simulink model "linearExtendedStateObserverModel"  (R2021a)
settings: Solver=VariableStepAuto  StartTime=0.0  StopTime=10.0  RelTol=1e-3
settings Model: Creator=krzys  LastModifiedBy=krzys

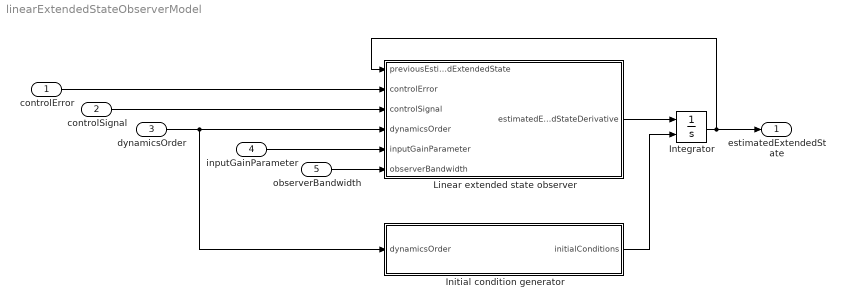
== system linearExtendedStateObserverModel ==
  controlError : Inport
  controlSignal : Inport  Port=2
  dynamicsOrder : Inport  Port=3
  inputGainParameter : Inport  Port=4
  observerBandwidth : Inport  Port=5
  Initial condition generator : MATLAB Function  TreatAsAtomicUnit=on
  Integrator : Integrator  InitialConditionSource=external
  Linear extended state observer : MATLAB Function  TreatAsAtomicUnit=on
  estimatedExtendedState : Outport
  wires:
  controlError/1 -> Linear extended state observer/2(controlError)
  controlSignal/1 -> Linear extended state observer/3(controlSignal)
  Linear extended state observer/1(estimatedExtendedStateDerivative) -> Integrator/1
  dynamicsOrder/1 -> Initial condition generator/1(dynamicsOrder), Linear extended state observer/4(dynamicsOrder)
  inputGainParameter/1 -> Linear extended state observer/5(inputGainParameter)
  observerBandwidth/1 -> Linear extended state observer/6(observerBandwidth)
  Initial condition generator/1(initialConditions) -> Integrator/2
  Integrator/1 -> Linear extended state observer/1(previousEstimatedExtendedState), estimatedExtendedState/1

== matlab function linearExtendedStateObserverModel/Initial condition generator ==
  data: dynamicsOrder input; initialConditions output
function initialConditions = fcn(dynamicsOrder)
    initialConditions = zeros(dynamicsOrder,1);
end

== matlab function linearExtendedStateObserverModel/Linear extended state observer ==
  data: previousEstimatedExtendedState input; controlError input; estimatedExtendedStateDerivative output; controlSignal input; dynamicsOrder input; inputGainParameter input; observerBandwidth input
function estimatedExtendedStateDerivative = fcn(previousEstimatedExtendedState,...
        controlError,...
        controlSignal,...
        dynamicsOrder,...
        inputGainParameter,...
        observerBandwidth)
    
    A = calculateObserverStateMatrix(dynamicsOrder);
    B = calculateObserverInputMatrix(inputGainParameter, dynamicsOrder);
    L = calculateObserverGainVector(observerBandwidth, dynamicsOrder);
    
    estimatedExtendedStateDerivative = A * previousEstimatedExtendedState +...
        B * controlSignal +...
        L * (controlError - previousEstimatedExtendedState(1));
end

function observerStateMatrix = calculateObserverStateMatrix(dynamicsOrder)
    observerStateMatrix = [zeros(dynamicsOrder,1), eye(dynamicsOrder);...
        zeros(1,dynamicsOrder+1)];
end

function observerInputMatrix = calculateObserverInputMatrix(inputGainParameter, dynamicsOrder)
    observerInputMatrix = [zeros(dynamicsOrder-1,1); -inputGainParameter; 0];
end

function observerGainVector = calculateObserverGainVector(observerBandwidth, dynamicsOrder)
    extendedGainVector = poly(-observerBandwidth * ones(1, dynamicsOrder+1))';
    observerGainVector = extendedGainVector(2:end);
end
